simulink model "QuadrotorModelv2017"  (R2017a)
settings: Solver=VariableStepAuto  StartTime=0.0  StopTime=60  RelTol=1e-3
values from neighbouring files (symbols this model uses):
  Ax = 0.1    [workspace.mat]
  Ay = 0.1    [workspace.mat]
  Az = 0.1    [workspace.mat]
  b = 3.59e-05    [workspace.mat]
  d = 2.081e-06    [workspace.mat]
  g = 9.81    [workspace.mat]
  Ixx = 0.00963    [workspace.mat]
  Iyy = 0.00963    [workspace.mat]
  Izz = 0.019    [workspace.mat]
  Jr = 0.04439    [workspace.mat]
  l = 0.24    [workspace.mat]
  m = 0.9928    [workspace.mat]
undefined symbols (not defined in the file or in its folder): sigbuilder_block
libraries: simulink x5
settings Model: Creator=cavci  LastModifiedBy=root
settings SFSimCC: SimUseLocalCustomCode=on
settings RTWCC: RTWUseLocalCustomCode=on

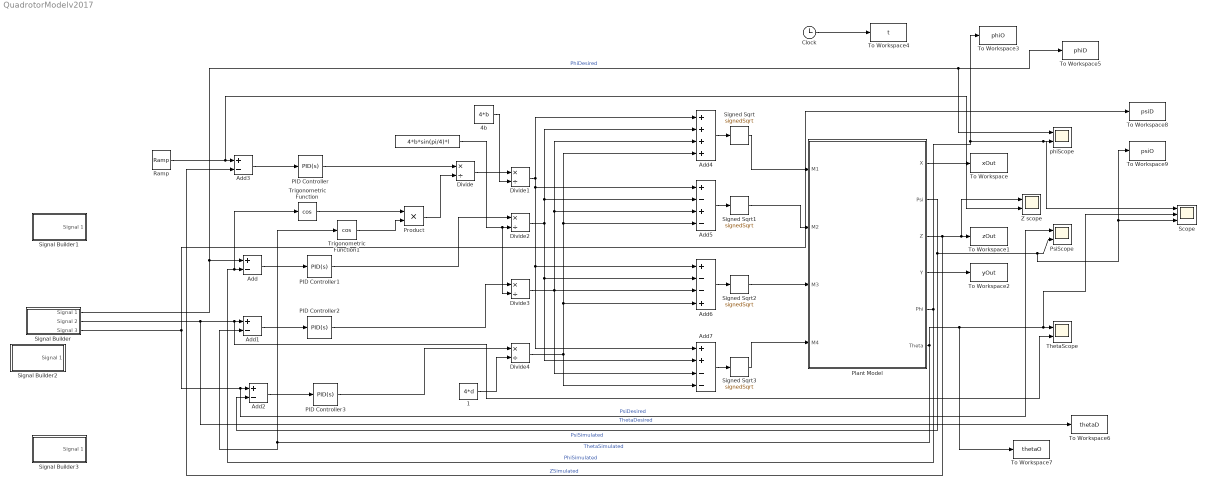
== system QuadrotorModelv2017 ==
  " " : Constant  Value=4*b*sin(pi/4)*l
  " 1" : Constant  Value=4*d
  "4b " : Constant  Value=4*b
  Add{,1..3} (4 alike) : Sum  Inputs=+-
  Add4 : Sum  Inputs=++++
  Add5 : Sum  Inputs=+-+-
  Add6 : Sum  Inputs=+--+
  Add7 : Sum  Inputs=++--
  Clock : Clock
  Divide{,1..4} (5 alike) : Product  Inputs=*/
  PID Controller : simulink/Continuous/PID Controller  Controller=PID  Form=Parallel  TimeDomain=Continuous-time  SampleTime=-1  IntegratorMethod=Forward Euler  FilterMethod=Forward Euler  ControllerParametersSource=internal  P=4.3  I=4.5  D=2  UseFilter=on  N=100  InitialConditionSource=internal  InitialConditionForIntegrator=0  InitialConditionForFilter=0  DifferentiatorICPrevScaledInput=0  ExternalReset=none  TrackingMode=off  Kt=1  LimitOutput=off  UpperSaturationLimit=inf  LowerSaturationLimit=-inf  LinearizeAsGain=on  AntiWindupMode=none  Kb=1  POutMin=[]  POutMax=[]  IOutMin=[]  IOutMax=[]  DOutMin=[]  DOutMax=[]  NOutMin=[]  NOutMax=[]  SumOutMin=[]  SumOutMax=[]  SaturationOutMin=[]  SaturationOutMax=[]  PParamMin=[]  PParamMax=[]  IParamMin=[]  IParamMax=[]  DParamMin=[]  DParamMax=[]  NParamMin=[]  NParamMax=[]  KbParamMin=[]  KbParamMax=[]  KtParamMin=[]  KtParamMax=[]  KbOutMin=[]  KbOutMax=[]  KtOutMin=[]  KtOutMax=[]  IntegratorOutMin=[]  IntegratorOutMax=[]  FilterOutMin=[]  FilterOutMax=[]  SumI1OutMin=[]  SumI1OutMax=[]  SumI2OutMin=[]  SumI2OutMax=[]  SumI3OutMin=[]  SumI3OutMax=[]  SumDOutMin=[]  SumDOutMax=[]  DifferentiatorOutMin=[]  DifferentiatorOutMax=[]  IntegratorContinuousStateAttributes=''  IntegratorStateMustResolveToSignalObject=off  IntegratorRTWStateStorageClass=Auto  FilterContinuousStateAttributes=''  FilterStateMustResolveToSignalObject=off  FilterRTWStateStorageClass=Auto
  PID Controller1 : simulink/Continuous/PID Controller  Controller=PID  Form=Parallel  TimeDomain=Continuous-time  SampleTime=-1  IntegratorMethod=Forward Euler  FilterMethod=Forward Euler  ControllerParametersSource=internal  P=0.006  I=0.000009  D=0.013  UseFilter=on  N=100  InitialConditionSource=internal  InitialConditionForIntegrator=0  InitialConditionForFilter=0  DifferentiatorICPrevScaledInput=0  ExternalReset=none  TrackingMode=off  Kt=1  LimitOutput=off  UpperSaturationLimit=inf  LowerSaturationLimit=-inf  LinearizeAsGain=on  AntiWindupMode=none  Kb=1  POutMin=[]  POutMax=[]  IOutMin=[]  IOutMax=[]  DOutMin=[]  DOutMax=[]  NOutMin=[]  NOutMax=[]  SumOutMin=[]  SumOutMax=[]  SaturationOutMin=[]  SaturationOutMax=[]  PParamMin=[]  PParamMax=[]  IParamMin=[]  IParamMax=[]  DParamMin=[]  DParamMax=[]  NParamMin=[]  NParamMax=[]  KbParamMin=[]  KbParamMax=[]  KtParamMin=[]  KtParamMax=[]  KbOutMin=[]  KbOutMax=[]  KtOutMin=[]  KtOutMax=[]  IntegratorOutMin=[]  IntegratorOutMax=[]  FilterOutMin=[]  FilterOutMax=[]  SumI1OutMin=[]  SumI1OutMax=[]  SumI2OutMin=[]  SumI2OutMax=[]  SumI3OutMin=[]  SumI3OutMax=[]  SumDOutMin=[]  SumDOutMax=[]  DifferentiatorOutMin=[]  DifferentiatorOutMax=[]  IntegratorContinuousStateAttributes=''  IntegratorStateMustResolveToSignalObject=off  IntegratorRTWStateStorageClass=Auto  FilterContinuousStateAttributes=''  FilterStateMustResolveToSignalObject=off  FilterRTWStateStorageClass=Auto
  PID Controller2 : simulink/Continuous/PID Controller  Controller=PID  Form=Parallel  TimeDomain=Continuous-time  SampleTime=-1  IntegratorMethod=Forward Euler  FilterMethod=Forward Euler  ControllerParametersSource=internal  P=0.006  I=0.000009  D=0.013  UseFilter=on  N=100  InitialConditionSource=internal  InitialConditionForIntegrator=0  InitialConditionForFilter=0  DifferentiatorICPrevScaledInput=0  ExternalReset=none  TrackingMode=off  Kt=1  LimitOutput=off  UpperSaturationLimit=inf  LowerSaturationLimit=-inf  LinearizeAsGain=on  AntiWindupMode=none  Kb=1  POutMin=[]  POutMax=[]  IOutMin=[]  IOutMax=[]  DOutMin=[]  DOutMax=[]  NOutMin=[]  NOutMax=[]  SumOutMin=[]  SumOutMax=[]  SaturationOutMin=[]  SaturationOutMax=[]  PParamMin=[]  PParamMax=[]  IParamMin=[]  IParamMax=[]  DParamMin=[]  DParamMax=[]  NParamMin=[]  NParamMax=[]  KbParamMin=[]  KbParamMax=[]  KtParamMin=[]  KtParamMax=[]  KbOutMin=[]  KbOutMax=[]  KtOutMin=[]  KtOutMax=[]  IntegratorOutMin=[]  IntegratorOutMax=[]  FilterOutMin=[]  FilterOutMax=[]  SumI1OutMin=[]  SumI1OutMax=[]  SumI2OutMin=[]  SumI2OutMax=[]  SumI3OutMin=[]  SumI3OutMax=[]  SumDOutMin=[]  SumDOutMax=[]  DifferentiatorOutMin=[]  DifferentiatorOutMax=[]  IntegratorContinuousStateAttributes=''  IntegratorStateMustResolveToSignalObject=off  IntegratorRTWStateStorageClass=Auto  FilterContinuousStateAttributes=''  FilterStateMustResolveToSignalObject=off  FilterRTWStateStorageClass=Auto
  PID Controller3 : simulink/Continuous/PID Controller  Controller=PID  Form=Parallel  TimeDomain=Continuous-time  SampleTime=-1  IntegratorMethod=Forward Euler  FilterMethod=Forward Euler  ControllerParametersSource=internal  P=0.01  I=0.0002  D=0.03  UseFilter=on  N=100  InitialConditionSource=internal  InitialConditionForIntegrator=0  InitialConditionForFilter=0  DifferentiatorICPrevScaledInput=0  ExternalReset=none  TrackingMode=off  Kt=1  LimitOutput=off  UpperSaturationLimit=inf  LowerSaturationLimit=-inf  LinearizeAsGain=on  AntiWindupMode=none  Kb=1  POutMin=[]  POutMax=[]  IOutMin=[]  IOutMax=[]  DOutMin=[]  DOutMax=[]  NOutMin=[]  NOutMax=[]  SumOutMin=[]  SumOutMax=[]  SaturationOutMin=[]  SaturationOutMax=[]  PParamMin=[]  PParamMax=[]  IParamMin=[]  IParamMax=[]  DParamMin=[]  DParamMax=[]  NParamMin=[]  NParamMax=[]  KbParamMin=[]  KbParamMax=[]  KtParamMin=[]  KtParamMax=[]  KbOutMin=[]  KbOutMax=[]  KtOutMin=[]  KtOutMax=[]  IntegratorOutMin=[]  IntegratorOutMax=[]  FilterOutMin=[]  FilterOutMax=[]  SumI1OutMin=[]  SumI1OutMax=[]  SumI2OutMin=[]  SumI2OutMax=[]  SumI3OutMin=[]  SumI3OutMax=[]  SumDOutMin=[]  SumDOutMax=[]  DifferentiatorOutMin=[]  DifferentiatorOutMax=[]  IntegratorContinuousStateAttributes=''  IntegratorStateMustResolveToSignalObject=off  IntegratorRTWStateStorageClass=Auto  FilterContinuousStateAttributes=''  FilterStateMustResolveToSignalObject=off  FilterRTWStateStorageClass=Auto
  Plant Model : Subsystem
  Product : Product
  PsiScope : Scope  NumInputPorts=2
  Ramp : simulink/Sources/Ramp  slope=1.5  start=0  X0=0
  Scope : Scope  NumInputPorts=3
  Signal Builder : Subsystem  Tag=STV Subsys  LoadFcn=sigbuilder_block('load');  StartFcn=sigbuilder_block('start');  StopFcn=sigbuilder_block('stop');  ClipboardFcn=sigbuilder_block('clipboard');  mask(Sigbuilder block){tuvar=[0:10]}
      mask help: Simulink:masks:SigbuilderBlock_MD
      mask init:
      | if ~strcmp(get_param(bdroot(gcbh),'SimulationStatus'),'stopped') tuvar = sigbuilder_block('maskInit'); end
      settings: CopyFcn=sigbuilder_block('copy');  DeleteFcn=sigbuilder_block('delete');  ModelCloseFcn=sigbuilder_block('modelClose');  PreSaveFcn=sigbuilder_block('preSave');  PauseFcn=sigbuilder_block('pause');  ContinueFcn=sigbuilder_block('continue');  NameChangeFcn=sigbuilder_block('namechange');  OpenFcn=sigbuilder_block('open',[273.897 181.856 497.32 325.856 ]);  CloseFcn=sigbuilder_block('close');
      mask Display: plot(0, 0, 100, 100,[2, 2, 32, 32, 2], [68, 8, 8, 68, 68],[32, 2], [38, 38], [32, 19, 2],[53, 60, 44], [32, 17, 17, 2],[16, 16, 31, 31]);txt = getActiveGroup(gcbh);text(2, 100, txt,'verticalAlignment', 'top');
  Signal Builder1 : Subsystem  Tag=STV Subsys  LoadFcn=sigbuilder_block('load');  StartFcn=sigbuilder_block('start');  StopFcn=sigbuilder_block('stop');  ClipboardFcn=sigbuilder_block('clipboard');  mask(Sigbuilder block){tuvar=[0:10]}
      mask help: Simulink:masks:SigbuilderBlock_MD
      mask init:
      | if ~strcmp(get_param(bdroot(gcbh),'SimulationStatus'),'stopped') tuvar = sigbuilder_block('maskInit'); end
      settings: CopyFcn=sigbuilder_block('copy');  DeleteFcn=sigbuilder_block('delete');  ModelCloseFcn=sigbuilder_block('modelClose');  PreSaveFcn=sigbuilder_block('preSave');  PauseFcn=sigbuilder_block('pause');  ContinueFcn=sigbuilder_block('continue');  NameChangeFcn=sigbuilder_block('namechange');  OpenFcn=sigbuilder_block('open',[502.515 236.784 676.206 311.753 ]);  CloseFcn=sigbuilder_block('close');
      mask Display: plot(0, 0, 100, 100,[2, 2, 32, 32, 2], [68, 8, 8, 68, 68],[32, 2], [38, 38], [32, 19, 2],[53, 60, 44], [32, 17, 17, 2],[16, 16, 31, 31]);txt = getActiveGroup(gcbh);text(2, 100, txt,'verticalAlignment', 'top');
  Signal Builder2 : Subsystem  Tag=STV Subsys  LoadFcn=sigbuilder_block('load');  StartFcn=sigbuilder_block('start');  StopFcn=sigbuilder_block('stop');  ClipboardFcn=sigbuilder_block('clipboard');  mask(Sigbuilder block){tuvar=[0:10]}
      mask help: Simulink:masks:SigbuilderBlock_MD
      mask init:
      | if ~strcmp(get_param(bdroot(gcbh),'SimulationStatus'),'stopped') tuvar = sigbuilder_block('maskInit'); end
      settings: CopyFcn=sigbuilder_block('copy');  DeleteFcn=sigbuilder_block('delete');  ModelCloseFcn=sigbuilder_block('modelClose');  PreSaveFcn=sigbuilder_block('preSave');  PauseFcn=sigbuilder_block('pause');  ContinueFcn=sigbuilder_block('continue');  NameChangeFcn=sigbuilder_block('namechange');  OpenFcn=sigbuilder_block('open',[385.979 141.773 646.515 332.536 ]);  CloseFcn=sigbuilder_block('close');
      mask Display: plot(0, 0, 100, 100,[2, 2, 32, 32, 2], [68, 8, 8, 68, 68],[32, 2], [38, 38], [32, 19, 2],[53, 60, 44], [32, 17, 17, 2],[16, 16, 31, 31]);txt = getActiveGroup(gcbh);text(2, 100, txt,'verticalAlignment', 'top');
  Signal Builder3 : Subsystem  Tag=STV Subsys  LoadFcn=sigbuilder_block('load');  StartFcn=sigbuilder_block('start');  StopFcn=sigbuilder_block('stop');  ClipboardFcn=sigbuilder_block('clipboard');  mask(Sigbuilder block){tuvar=[0:10]}
      mask help: Simulink:masks:SigbuilderBlock_MD
      mask init:
      | if ~strcmp(get_param(bdroot(gcbh),'SimulationStatus'),'stopped') tuvar = sigbuilder_block('maskInit'); end
      settings: CopyFcn=sigbuilder_block('copy');  DeleteFcn=sigbuilder_block('delete');  ModelCloseFcn=sigbuilder_block('modelClose');  PreSaveFcn=sigbuilder_block('preSave');  PauseFcn=sigbuilder_block('pause');  ContinueFcn=sigbuilder_block('continue');  NameChangeFcn=sigbuilder_block('namechange');  OpenFcn=sigbuilder_block('open',[389.691 135.093 624.247 348.124 ]);  CloseFcn=sigbuilder_block('close');
      mask Display: plot(0, 0, 100, 100,[2, 2, 32, 32, 2], [68, 8, 8, 68, 68],[32, 2], [38, 38], [32, 19, 2],[53, 60, 44], [32, 17, 17, 2],[16, 16, 31, 31]);txt = getActiveGroup(gcbh);text(2, 100, txt,'verticalAlignment', 'top');
  Signed Sqrt{,1..3} (4 alike) : Sqrt  Operator=signedSqrt  SaturateOnIntegerOverflow=on
  ThetaScope : Scope  NumInputPorts=2
  To Workspace : ToWorkspace  VariableName=xOut  SaveFormat=Timeseries  SampleTime=-1
  To Workspace1 : ToWorkspace  VariableName=zOut  SaveFormat=Timeseries  SampleTime=-1
  To Workspace2 : ToWorkspace  VariableName=yOut  SaveFormat=Timeseries  SampleTime=-1
  To Workspace3 : ToWorkspace  VariableName=phiO  SampleTime=-1
  To Workspace4 : ToWorkspace  VariableName=t  SampleTime=-1
  To Workspace5 : ToWorkspace  VariableName=phiD  SampleTime=-1
  To Workspace6 : ToWorkspace  VariableName=thetaD  SampleTime=-1
  To Workspace7 : ToWorkspace  VariableName=thetaO  SampleTime=-1
  To Workspace8 : ToWorkspace  VariableName=psiD  SampleTime=-1
  To Workspace9 : ToWorkspace  VariableName=psiO  SampleTime=-1
  Trigonometric Function : Trigonometry  Operator=cos
  Trigonometric Function1 : Trigonometry  Operator=cos
  Z scope : Scope  NumInputPorts=2
  phiScope : Scope  NumInputPorts=2
  wires:
  Signed Sqrt3/1 -> Plant Model/4(M4)
  Clock/1 -> To Workspace4/1
  Divide4/1 -> Add7/4, Add5/4, Add4/4, Add6/4
  Divide2/1 -> Add6/2, Add7/2, Add4/2, Add5/2
  Signal Builder/3(Signal 3) -> PsiScope/1, Add2/1, To Workspace8/1  "PsiDesired"
  Ramp/1 -> Z scope/2, Add3/1
  Plant Model/2(Psi) -> Scope/3, To Workspace9/1, PsiScope/2, Add2/2  "PsiSimulated"
  Trigonometric Function1/1 -> Product/2
  PID Controller3/1 -> Divide4/1
  Plant Model/6(Theta) -> To Workspace7/1, Scope/2, ThetaScope/1, Add1/2, Trigonometric Function1/1  "ThetaSimulated"
  Add1/1 -> PID Controller2/1
  PID Controller2/1 -> Divide3/1
  Signal Builder/2(Signal 2) -> To Workspace6/1, ThetaScope/2, Add1/1  "ThetaDesired"
  Add4/1 -> Signed Sqrt/1
  Add/1 -> PID Controller1/1
  Signed Sqrt2/1 -> Plant Model/3(M3)
  "4b "/1 -> Divide1/2
  Plant Model/1(X) -> To Workspace/1
  " "/1 -> Divide3/2, Divide2/2
  PID Controller/1 -> Divide/1
  Signed Sqrt1/1 -> Plant Model/2("M2 ")
  " 1"/1 -> Divide4/2
  Plant Model/5(Phi) -> Scope/1, phiScope/2, To Workspace3/1, Trigonometric Function/1, Add/2  "PhiSimulated"
  Divide1/1 -> Add7/1, Add6/1, Add5/1, Add4/1
  Signed Sqrt/1 -> Plant Model/1("M1 ")
  Signal Builder/1(Signal 1) -> Add/1, To Workspace5/1, phiScope/1  "PhiDesired"
  Product/1 -> Divide/2
  Plant Model/4(Y) -> To Workspace2/1
  Trigonometric Function/1 -> Product/1
  Add6/1 -> Signed Sqrt2/1
  Divide3/1 -> Add7/3, Add4/3, Add5/3, Add6/3
  Add3/1 -> PID Controller/1
  PID Controller1/1 -> Divide2/1
  Divide/1 -> Divide1/1
  Add7/1 -> Signed Sqrt3/1
  Add2/1 -> PID Controller3/1
  Plant Model/3(Z) -> Z scope/1, To Workspace1/1, Add3/2  "ZSimulated"
  Add5/1 -> Signed Sqrt1/1

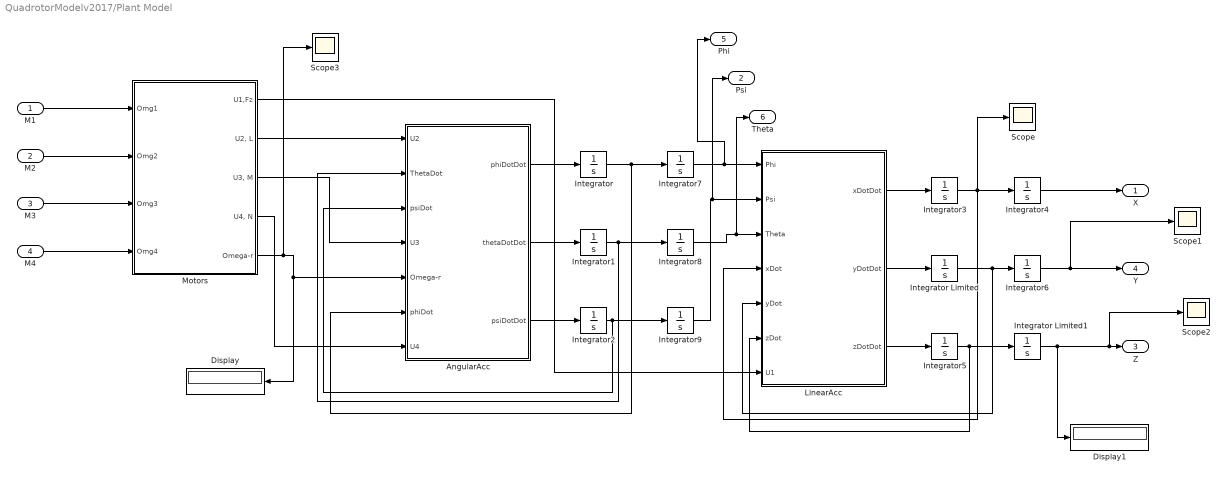
== system QuadrotorModelv2017/Plant Model ==
  "M1 " : Inport
  "M2 " : Inport  Port=2
  M3 : Inport  Port=3
  M4 : Inport  Port=4
  AngularAcc : Subsystem
  Display : Display
  Display1 : Display
  Integrator{,1..6} (7 alike) : Integrator
  Integrator Limited : Integrator  LimitOutput=on  UpperSaturationLimit=1  LowerSaturationLimit=0
  Integrator Limited1 : Integrator  LimitOutput=on  LowerSaturationLimit=0
  Integrator7 : Integrator  WrapState=on
  Integrator8 : Integrator  WrapState=on
  Integrator9 : Integrator  WrapState=on
  "LinearAcc " : Subsystem
  "Motors " : Subsystem
  Scope{,1..3} (4 alike) : Scope
  X : Outport
  Psi : Outport  Port=2
  Z : Outport  Port=3
  Y : Outport  Port=4
  Phi : Outport  Port=5
  Theta : Outport  Port=6
  wires:
  AngularAcc/3(psiDotDot) -> Integrator2/1
  "M1 "/1 -> "Motors "/1(Omg1)
  "Motors "/5(Omega-r) -> Scope3/1, Display/1, AngularAcc/5(Omega-r)
  AngularAcc/1(phiDotDot) -> Integrator/1
  M3/1 -> "Motors "/3("Omg3 ")
  Integrator3/1 -> "LinearAcc "/4("xDot "), Integrator4/1, Scope/1
  "Motors "/3("U3, M") -> AngularAcc/4("U3 ")
  AngularAcc/2(thetaDotDot) -> Integrator1/1
  Integrator5/1 -> "LinearAcc "/6(zDot), Integrator Limited1/1
  M4/1 -> "Motors "/4("Omg4 ")
  "M2 "/1 -> "Motors "/2(Omg2)
  "LinearAcc "/1(xDotDot) -> Integrator3/1
  Integrator1/1 -> Integrator8/1, AngularAcc/2(ThetaDot)
  "Motors "/4("U4, N") -> AngularAcc/7(U4)
  "Motors "/2("U2, L") -> AngularAcc/1(U2)
  Integrator/1 -> Integrator7/1, AngularAcc/6("phiDot ")
  Integrator2/1 -> Integrator9/1, AngularAcc/3("psiDot ")
  "LinearAcc "/3(zDotDot) -> Integrator5/1
  Integrator4/1 -> X/1
  "LinearAcc "/2(yDotDot) -> Integrator Limited/1
  Integrator Limited/1 -> "LinearAcc "/5(yDot), Integrator6/1
  Integrator6/1 -> Scope1/1, Y/1
  Integrator Limited1/1 -> Display1/1, Scope2/1, Z/1
  Integrator7/1 -> Phi/1, "LinearAcc "/1(Phi)
  Integrator8/1 -> Theta/1, "LinearAcc "/3(Theta)
  Integrator9/1 -> "LinearAcc "/2(Psi), Psi/1
  "Motors "/1("U1,Fz ") -> "LinearAcc "/7(U1)

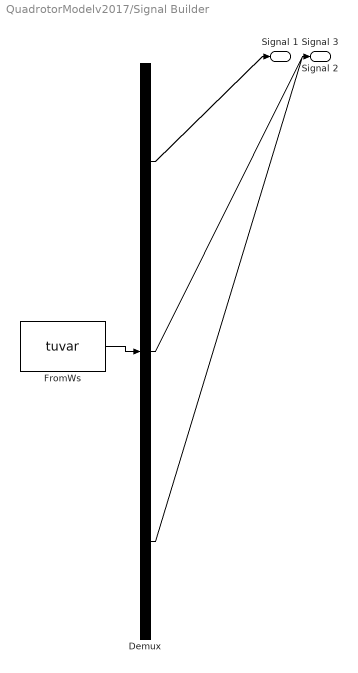
== system QuadrotorModelv2017/Signal Builder ==
  Demux : Demux  Tag=STV Demux  Outputs=3
  FromWs : FromWorkspace  Tag=STV FromWs  VariableName=tuvar  SampleTime=0
      SigBuilderData=|
      | common.afterFinalStr = 'Extrapolate'
      | common.sampleTime = 0
      | dataSet.timeRange = [0 60]
      | dataSet.name = 'Group 1'
      | sbobj.Groups.Name = 'Group 1'
      | sbobj.Groups.Signals(1).Name = 'Signal 1'
      | sbobj.Groups.Signals(1).XData = [0 10 10 20 20 50 50 60]
      | sbobj.Groups.Signals(1).YData = [0 0 0.2 0.2 0 0 0.2 0.2]
      | sbobj.Groups.Signals(2).Name = 'Signal 2'
      | sbobj.Groups.Signals(2).XData = [0 30 30 40 40 60]
      | sbobj.Groups.Signals(2).YData = [0 0 0.2 0.2 0 0]
      | sbobj.Groups.Signals(3).Name = 'Signal 3'
      | sbobj.Groups.Signals(3).XData = [0 5 5 10 10 60]
      | sbobj.Groups.Signals(3).YData = [0 0 0.5 0.5 0 0]
      | sbobj.Groups.TimeRange = [0 60]
  Signal 1 : Outport  Tag=STV Outport
  Signal 2 : Outport  Tag=STV Outport  Port=2
  Signal 3 : Outport  Tag=STV Outport  Port=3
  wires:
  FromWs/1 -> Demux/1
  Demux/1 -> Signal 1/1
  Demux/2 -> Signal 2/1
  Demux/3 -> Signal 3/1

== system QuadrotorModelv2017/Signal Builder1 ==
  Demux : Demux  Tag=STV Demux  Outputs=1
  FromWs : FromWorkspace  Tag=STV FromWs  VariableName=tuvar  SampleTime=0
      SigBuilderData=|
      | common.afterFinalStr = 'Extrapolate'
      | common.sampleTime = 0
      | dataSet.timeRange = [0 60]
      | dataSet.name = 'Group 1'
      | sbobj.Groups.Name = 'Group 1'
      | sbobj.Groups.Signals.Name = 'Signal 1'
      | sbobj.Groups.Signals.XData = [0 10 10 20 20 50 50 60]
      | sbobj.Groups.Signals.YData = [0 0 0.2 0.2 0 0 0.2 0.2]
      | sbobj.Groups.TimeRange = [0 60]
  Signal 1 : Outport  Tag=STV Outport
  wires:
  FromWs/1 -> Demux/1
  Demux/1 -> Signal 1/1

== system QuadrotorModelv2017/Signal Builder2 ==
  Demux : Demux  Tag=STV Demux  Outputs=1
  FromWs : FromWorkspace  Tag=STV FromWs  VariableName=tuvar  SampleTime=0
      SigBuilderData=|
      | common.afterFinalStr = 'Extrapolate'
      | common.sampleTime = 0
      | dataSet.timeRange = [0 60]
      | dataSet.name = 'Group 1'
      | sbobj.Groups.Name = 'Group 1'
      | sbobj.Groups.Signals.Name = 'Signal 1'
      | sbobj.Groups.Signals.XData = [0 30 30 40 40 60]
      | sbobj.Groups.Signals.YData = [0 0 0.2 0.2 0 0]
      | sbobj.Groups.TimeRange = [0 60]
  Signal 1 : Outport  Tag=STV Outport
  wires:
  Demux/1 -> Signal 1/1
  FromWs/1 -> Demux/1

== system QuadrotorModelv2017/Signal Builder3 ==
  Demux : Demux  Tag=STV Demux  Outputs=1
  FromWs : FromWorkspace  Tag=STV FromWs  VariableName=tuvar  SampleTime=0
      SigBuilderData=|
      | common.afterFinalStr = 'Extrapolate'
      | common.sampleTime = 0
      | dataSet.timeRange = [0 60]
      | dataSet.name = 'Group 1'
      | sbobj.Groups.Name = 'Group 1'
      | sbobj.Groups.Signals.Name = 'Signal 1'
      | sbobj.Groups.Signals.XData = [0 5 5 11 11 60]
      | sbobj.Groups.Signals.YData = [0 0 0.5 0.5 0 0.006]
      | sbobj.Groups.TimeRange = [0 60]
  Signal 1 : Outport  Tag=STV Outport
  wires:
  Demux/1 -> Signal 1/1
  FromWs/1 -> Demux/1

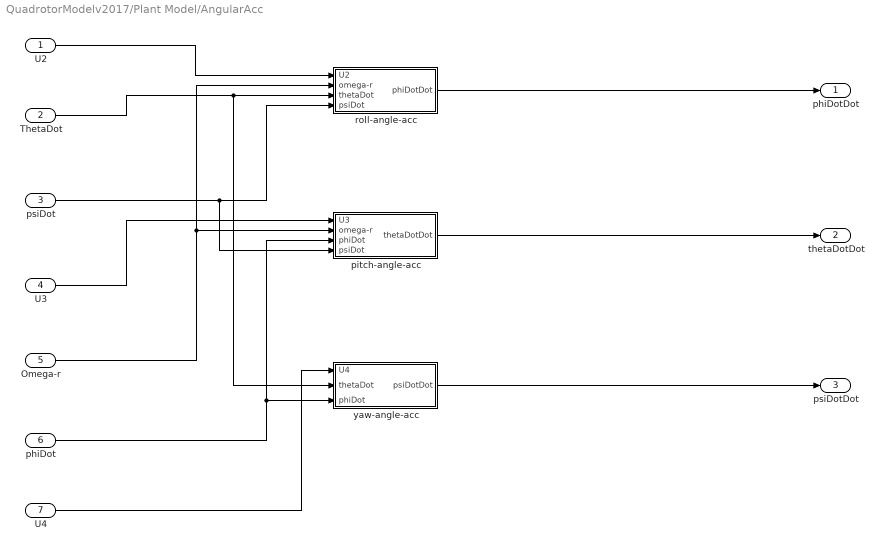
== system QuadrotorModelv2017/Plant Model/AngularAcc ==
  U2 : Inport
  ThetaDot : Inport  Port=2
  "psiDot " : Inport  Port=3
  "U3 " : Inport  Port=4
  Omega-r : Inport  Port=5
  "phiDot " : Inport  Port=6
  U4 : Inport  Port=7
  pitch-angle-acc : Subsystem
  roll-angle-acc : Subsystem
  yaw-angle-acc : Subsystem
  phiDotDot : Outport
  thetaDotDot : Outport  Port=2
  psiDotDot : Outport  Port=3
  wires:
  roll-angle-acc/1(phiDotDot) -> phiDotDot/1
  pitch-angle-acc/1(thetaDotDot) -> thetaDotDot/1
  yaw-angle-acc/1(psiDotDot) -> psiDotDot/1
  U2/1 -> roll-angle-acc/1(U2)
  Omega-r/1 -> pitch-angle-acc/2(omega-r), roll-angle-acc/2(omega-r)
  ThetaDot/1 -> yaw-angle-acc/2(thetaDot), roll-angle-acc/3(thetaDot)
  "psiDot "/1 -> pitch-angle-acc/4(psiDot), roll-angle-acc/4("psiDot ")
  "U3 "/1 -> pitch-angle-acc/1(U3)
  "phiDot "/1 -> yaw-angle-acc/3(phiDot), pitch-angle-acc/3(phiDot)
  U4/1 -> yaw-angle-acc/1(U4)

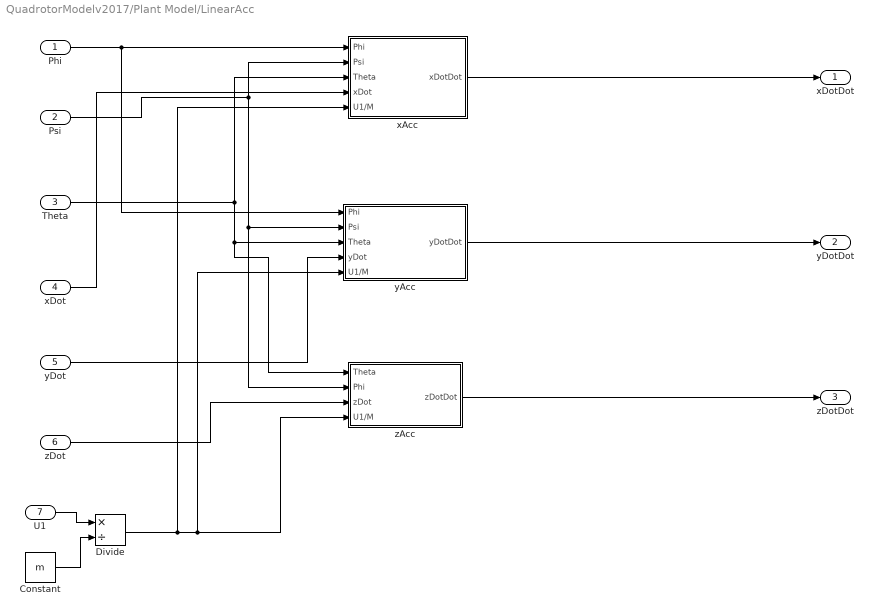
== system QuadrotorModelv2017/Plant Model/LinearAcc  ==
  Phi : Inport
  Psi : Inport  Port=2
  Theta : Inport  Port=3
  "xDot " : Inport  Port=4
  yDot : Inport  Port=5
  zDot : Inport  Port=6
  U1 : Inport  Port=7
  Constant : Constant  Value=m
  Divide : Product  Inputs=*/
  xAcc : Subsystem
  "yAcc " : Subsystem
  zAcc : Subsystem
  xDotDot : Outport
  yDotDot : Outport  Port=2
  zDotDot : Outport  Port=3
  wires:
  zDot/1 -> zAcc/3("zDot ")
  Theta/1 -> xAcc/3(Theta), "yAcc "/3(Theta), zAcc/1(Theta)
  Psi/1 -> "yAcc "/2(Psi), zAcc/2(Phi), xAcc/2(Psi)
  yDot/1 -> "yAcc "/4("yDot ")
  Phi/1 -> "yAcc "/1(Phi), xAcc/1(Phi)
  zAcc/1(zDotDot) -> zDotDot/1
  "yAcc "/1(yDotDot) -> yDotDot/1
  xAcc/1(xDotDot) -> xDotDot/1
  "xDot "/1 -> xAcc/4("xDot ")
  Constant/1 -> Divide/2
  U1/1 -> Divide/1
  Divide/1 -> xAcc/5(U1/M), "yAcc "/5(U1/M), zAcc/4("U1/M ")

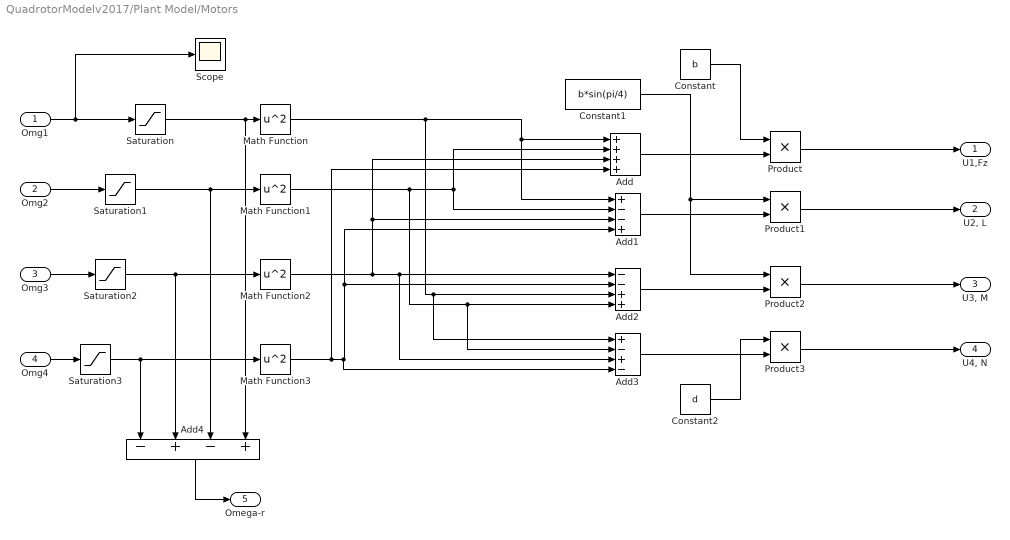
== system QuadrotorModelv2017/Plant Model/Motors  ==
  Omg1 : Inport
  Omg2 : Inport  Port=2
  "Omg3 " : Inport  Port=3
  "Omg4 " : Inport  Port=4
  Add : Sum  Inputs=++++
  Add1 : Sum  Inputs=+--+
  Add2 : Sum  Inputs=--++
  Add3 : Sum  Inputs=+-+-
  Add4 : Sum  Inputs=-+-+
  Constant : Constant  Value=b
  Constant1 : Constant  Value=b*sin(pi/4)
  Constant2 : Constant  Value=d
  Math Function{,1..3} (4 alike) : Math  Operator=square  SaturateOnIntegerOverflow=on
  Product{,1..3} (4 alike) : Product
  Saturation{,1..3} (4 alike) : Saturate  UpperLimit=1472  LowerLimit=0
  Scope : Scope
  "U1,Fz " : Outport
  "U2, L" : Outport  Port=2
  "U3, M" : Outport  Port=3
  "U4, N" : Outport  Port=4
  Omega-r : Outport  Port=5
  wires:
  Math Function/1 -> Add3/1, Add2/3, Add1/1, Add/1
  Math Function1/1 -> Add3/2, Add2/4, Add1/2, Add/2
  Math Function2/1 -> Add/3, Add1/3, Add3/3, Add2/1
  Math Function3/1 -> Add/4, Add3/4, Add2/2, Add1/4
  Constant/1 -> Product/1
  Product/1 -> "U1,Fz "/1
  Product1/1 -> "U2, L"/1
  Product2/1 -> "U3, M"/1
  Product3/1 -> "U4, N"/1
  Add/1 -> Product/2
  Constant1/1 -> Product2/1, Product1/1
  Add1/1 -> Product1/2
  Add2/1 -> Product2/2
  Add3/1 -> Product3/2
  Constant2/1 -> Product3/1
  Add4/1 -> Omega-r/1
  Omg1/1 -> Saturation/1, Scope/1
  Omg2/1 -> Saturation1/1
  "Omg3 "/1 -> Saturation2/1
  "Omg4 "/1 -> Saturation3/1
  Saturation/1 -> Add4/4, Math Function/1
  Saturation1/1 -> Add4/3, Math Function1/1
  Saturation2/1 -> Math Function2/1, Add4/2
  Saturation3/1 -> Math Function3/1, Add4/1

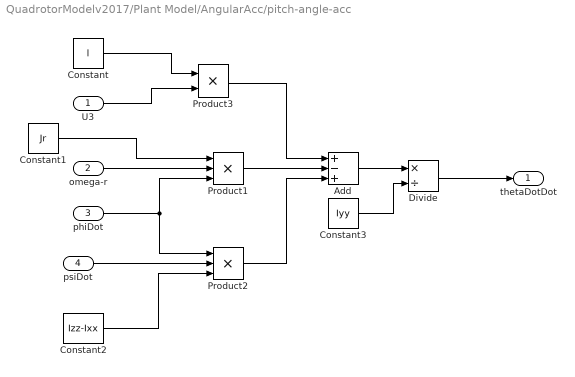
== system QuadrotorModelv2017/Plant Model/AngularAcc/pitch-angle-acc ==
  U3 : Inport
  omega-r : Inport  Port=2
  phiDot : Inport  Port=3
  psiDot : Inport  Port=4
  Add : Sum  Inputs=+-+
  Constant : Constant  Value=l
  Constant1 : Constant  Value=Jr
  Constant2 : Constant  Value=Izz-Ixx
  Constant3 : Constant  Value=Iyy
  Divide : Product  Inputs=*/
  Product1 : Product  Inputs=3
  Product2 : Product  Inputs=3
  Product3 : Product
  thetaDotDot : Outport
  wires:
  Constant/1 -> Product3/1
  Constant1/1 -> Product1/1
  omega-r/1 -> Product1/2
  phiDot/1 -> Product2/1, Product1/3
  psiDot/1 -> Product2/2
  Constant2/1 -> Product2/3
  Product1/1 -> Add/2
  Product2/1 -> Add/3
  Add/1 -> Divide/1
  Constant3/1 -> Divide/2
  Divide/1 -> thetaDotDot/1
  U3/1 -> Product3/2
  Product3/1 -> Add/1

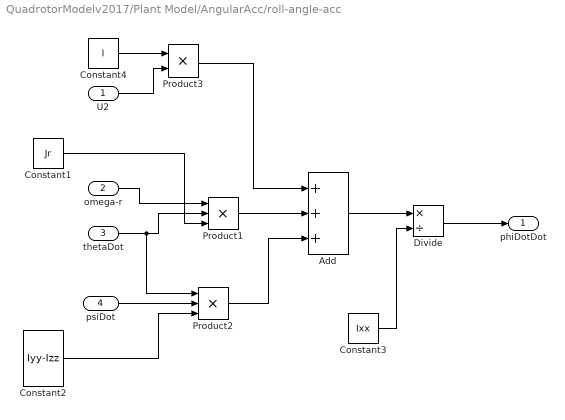
== system QuadrotorModelv2017/Plant Model/AngularAcc/roll-angle-acc ==
  U2 : Inport
  omega-r : Inport  Port=2
  thetaDot : Inport  Port=3
  "psiDot " : Inport  Port=4
  Add : Sum  Inputs=+++
  Constant1 : Constant  Value=Jr
  Constant2 : Constant  Value=Iyy-Izz
  Constant3 : Constant  Value=Ixx
  Constant4 : Constant  Value=l
  Divide : Product  Inputs=*/
  Product1 : Product  Inputs=3
  Product2 : Product  Inputs=3
  Product3 : Product
  phiDotDot : Outport
  wires:
  omega-r/1 -> Product1/1
  thetaDot/1 -> Product2/1, Product1/2
  Constant1/1 -> Product1/3
  "psiDot "/1 -> Product2/2
  Constant2/1 -> Product2/3
  U2/1 -> Product3/2
  Product1/1 -> Add/2
  Product2/1 -> Add/3
  Add/1 -> Divide/1
  Constant3/1 -> Divide/2
  Divide/1 -> phiDotDot/1
  Constant4/1 -> Product3/1
  Product3/1 -> Add/1

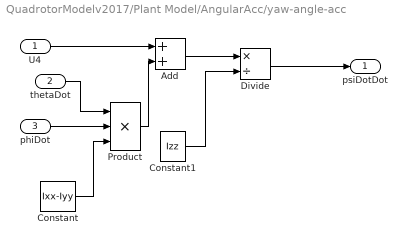
== system QuadrotorModelv2017/Plant Model/AngularAcc/yaw-angle-acc ==
  U4 : Inport
  thetaDot : Inport  Port=2
  phiDot : Inport  Port=3
  Add : Sum
  Constant : Constant  Value=Ixx-Iyy
  Constant1 : Constant  Value=Izz
  Divide : Product  Inputs=*/
  Product : Product  Inputs=3
  psiDotDot : Outport
  wires:
  Constant/1 -> Product/3
  phiDot/1 -> Product/2
  thetaDot/1 -> Product/1
  U4/1 -> Add/1
  Product/1 -> Add/2
  Add/1 -> Divide/1
  Constant1/1 -> Divide/2
  Divide/1 -> psiDotDot/1

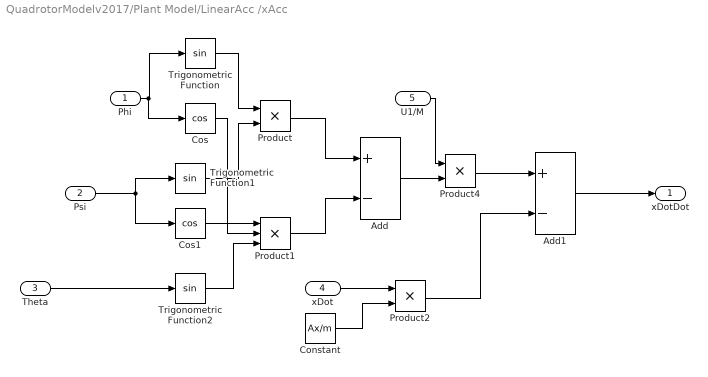
== system QuadrotorModelv2017/Plant Model/LinearAcc /xAcc ==
  Phi : Inport
  Psi : Inport  Port=2
  Theta : Inport  Port=3
  "xDot " : Inport  Port=4
  U1/M : Inport  Port=5
  Add : Sum  Inputs=+-
  Add1 : Sum  Inputs=+-
  Constant : Constant  Value=Ax/m
  Cos : Trigonometry  Operator=cos
  Cos1 : Trigonometry  Operator=cos
  Product : Product
  Product1 : Product  Inputs=3
  Product2 : Product
  Product4 : Product
  Trigonometric Function : Trigonometry
  Trigonometric Function1 : Trigonometry
  Trigonometric Function2 : Trigonometry
  xDotDot : Outport
  wires:
  Phi/1 -> Cos/1, Trigonometric Function/1
  Psi/1 -> Cos1/1, Trigonometric Function1/1
  Theta/1 -> Trigonometric Function2/1
  Trigonometric Function/1 -> Product/1
  Trigonometric Function1/1 -> Product/2
  Product/1 -> Add/1
  Product1/1 -> Add/2
  Cos1/1 -> Product1/1
  Cos/1 -> Product1/2
  Trigonometric Function2/1 -> Product1/3
  "xDot "/1 -> Product2/1
  Constant/1 -> Product2/2
  Add/1 -> Product4/2
  U1/M/1 -> Product4/1
  Product4/1 -> Add1/1
  Product2/1 -> Add1/2
  Add1/1 -> xDotDot/1

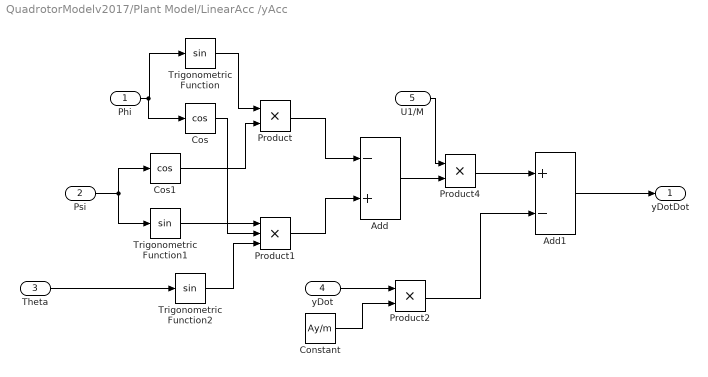
== system QuadrotorModelv2017/Plant Model/LinearAcc /yAcc  ==
  Phi : Inport
  Psi : Inport  Port=2
  Theta : Inport  Port=3
  "yDot " : Inport  Port=4
  U1/M : Inport  Port=5
  Add : Sum  Inputs=-+
  Add1 : Sum  Inputs=+-
  Constant : Constant  Value=Ay/m
  Cos : Trigonometry  Operator=cos
  Cos1 : Trigonometry  Operator=cos
  Product : Product
  Product1 : Product  Inputs=3
  Product2 : Product
  Product4 : Product
  Trigonometric Function : Trigonometry
  Trigonometric Function1 : Trigonometry
  Trigonometric Function2 : Trigonometry
  yDotDot : Outport
  wires:
  "yDot "/1 -> Product2/1
  Product/1 -> Add/1
  Product2/1 -> Add1/2
  Product4/1 -> Add1/1
  Add/1 -> Product4/2
  Phi/1 -> Cos/1, Trigonometric Function/1
  Trigonometric Function/1 -> Product/1
  Product1/1 -> Add/2
  Theta/1 -> Trigonometric Function2/1
  U1/M/1 -> Product4/1
  Add1/1 -> yDotDot/1
  Constant/1 -> Product2/2
  Cos/1 -> Product1/2
  Trigonometric Function2/1 -> Product1/3
  Psi/1 -> Trigonometric Function1/1, Cos1/1
  Cos1/1 -> Product/2
  Trigonometric Function1/1 -> Product1/1

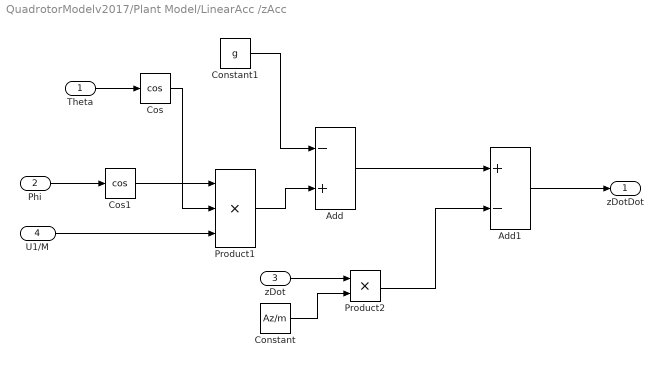
== system QuadrotorModelv2017/Plant Model/LinearAcc /zAcc ==
  Theta : Inport
  Phi : Inport  Port=2
  "zDot " : Inport  Port=3
  "U1/M " : Inport  Port=4
  Add : Sum  Inputs=-+
  Add1 : Sum  Inputs=+-
  Constant : Constant  Value=Az/m
  Constant1 : Constant  Value=g
  Cos : Trigonometry  Operator=cos
  Cos1 : Trigonometry  Operator=cos
  Product1 : Product  Inputs=3
  Product2 : Product
  zDotDot : Outport
  wires:
  Phi/1 -> Cos1/1
  Cos/1 -> Product1/2
  Theta/1 -> Cos/1
  Add1/1 -> zDotDot/1
  Product1/1 -> Add/2
  Add/1 -> Add1/1
  Constant/1 -> Product2/2
  Product2/1 -> Add1/2
  Cos1/1 -> Product1/1
  "zDot "/1 -> Product2/1
  "U1/M "/1 -> Product1/3
  Constant1/1 -> Add/1
